simulink model "quadcopter_model_c_NewtonEuler"  (Simulink 10.1)
settings: Solver=ode3  StartTime=0.0  StopTime=100  FixedStep=inner_h  RelTol=1e-3  EnableMultiTasking=on
values from neighbouring files (symbols this model uses):
  A = [9.2e-07 9.1e-07 1.03e-06]    [dataset.mat]    (also in initiateVars.m = [0.92e-6; system_workspace.mat; system_workspace_ayk.mat)
  g = 9.81    [dataset.mat]    (also in initiateVars.m; system_workspace.mat; system_workspace_ayk.mat)
  I = eye(length(x_pred))    [MCKF.m]    (also in dataset.mat = [1.66e-05 1.66e-05 2.93e-05]; initiateVars.m = [1.66e-5; system_workspace.mat = [1.66e-05 1.66e-05 2.93e-05]; system_workspace_ayk.mat = [1.66e-05 1.66e-05 2.93e-05])
  m = 0.027    [dataset.mat]    (also in initiateVars.m; system_workspace.mat; system_workspace_ayk.mat)
libraries: sharedutil x1
settings Model: Creator=Daniel  LastModifiedBy=fethi
settings DataIOCC: LimitDataPoints=on  SaveFormat=Dataset
settings DebuggingCC: UnderspecifiedInitializationDetection=Simplified  MergeDetectMultiDrivingBlocksExec=error  AllowSymbolicDim=off  SFExecutionAtInitializationDiag=warning
settings HardwareCC: ProdBitPerPointer=64  ProdBitPerSizeT=64  ProdBitPerPtrDiffT=64  ProdLargestAtomicFloat=Float  ProdIntDivRoundTo=Zero  ProdEndianess=LittleEndian  ProdWordSize=64  ProdHWDeviceType=Intel->x86-64 (Windows64)
settings GRTTargetCC: CombineOutputUpdateFcns=on  GRTInterface=off

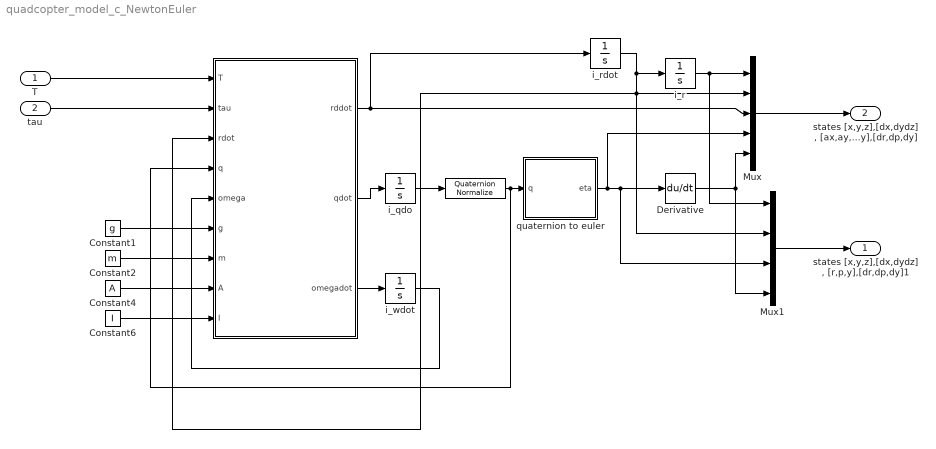
== system quadcopter_model_c_NewtonEuler ==
  T : Inport  PortDimensions=1
  tau : Inport  Port=2  PortDimensions=3
  " " : MATLAB Function  TreatAsAtomicUnit=on
  "  " : sharedutil/Quaternion Normalize  aMode=aMode
      settings: SourceProductBaseCode=AE,PW,MT,VE,VP
  Constant1 : Constant  Value=g
  Constant2 : Constant  Value=m
  Constant4 : Constant  Value=A
  Constant6 : Constant  Value=I
  Derivative : Derivative
  Mux : Mux  Inputs=5
  Mux1 : Mux
  i_qdo : Integrator  InitialCondition=[1; 0; 0; 0]
  i_r : Integrator  InitialCondition=[0.2 0.2 0]'
  i_rdot : Integrator  InitialCondition=[0; 0; 0]
  i_wdot : Integrator  InitialCondition=[0; 0; 0]
  quaternion to euler : MATLAB Function  TreatAsAtomicUnit=on
  "states [x,y,z],[dx,dydz], [r,p,y],[dr,dp,dy]1" : Outport  PortDimensions=12  VectorParamsAs1DForOutWhenUnconnected=off
  "states [x,y,z],[dx,dydz], [ax,ay,az],[r,p,y],[dr,dp,dy]" : Outport  Port=2  PortDimensions=15  VectorParamsAs1DForOutWhenUnconnected=off
  wires:
  " "/2(qdot) -> i_qdo/1
  " "/1(rddot) -> i_rdot/1, Mux/3
  i_r/1 -> Mux/1, Mux1/1
  T/1 -> " "/1(T)
  i_rdot/1 -> " "/3(rdot), Mux1/2, Mux/2, i_r/1
  tau/1 -> " "/2(tau)
  " "/3(omegadot) -> i_wdot/1
  Constant1/1 -> " "/6(g)
  Constant2/1 -> " "/7(m)
  Constant4/1 -> " "/8(A)
  Constant6/1 -> " "/9(I)
  i_wdot/1 -> " "/5(omega)
  i_qdo/1 -> "  "/1
  "  "/1 -> " "/4(q), quaternion to euler/1(q)
  quaternion to euler/1(eta) -> Mux/4, Mux1/3, Derivative/1
  Derivative/1 -> Mux/5, Mux1/4
  Mux/1 -> "states [x,y,z],[dx,dydz], [ax,ay,az],[r,p,y],[dr,dp,dy]"/1
  Mux1/1 -> "states [x,y,z],[dx,dydz], [r,p,y],[dr,dp,dy]1"/1

== matlab function   ==
  data: T input double; tau input double; rddot output double; rdot input double; q input double; omega input double; qdot output double; g input double; m input double; A input double; I input double; omegadot output double
function [ rddot,qdot,omegadot] = quad_acceleration(T, tau, rdot, q, omega, g, m, A, I)

    qw = q(1); qx = q(2); qy = q(3); qz = q(4); qv = q(2:4);
    omegaw = 0; omegav = omega;
    
    % Gravity acceleration
    Ga = -g * [0; 0; 1];

    % TODO write rotation
    angM = [2*(qx*qz + qw*qy);
            2*(qy*qz - qw*qx);
            qw.^2 - qx.^2 - qy.^2 + qz.^2];

    Ta = (T/m) .* angM;

    % Drag
    Aa = -1/m * diag(A) * rdot;
    rddot = Ga + Ta + Aa;
    
    % Define the C-matrix as (19)
    J = diag(I);
    qcross = [0, -qz, qy; qz, 0, -qx; -qy, qx, 0];
    qdot = 0.5.*(eye(4)*qw  + [0, -qv';qv, qcross])*[0; omegav];
    omegadot = J\(tau - cross(omegav, J*omegav));
    
%     R = [qw^2+qx^2+qy^2+qz^2, 2*(qx*qy-qw*qz)    , 2*(qx*qz+qw*qy);
%          2*(qx*qy+qw*qz)    , qw^2-qx^2+qy^2-qz^2, 2*(qy*qz-qw*qx);
%          2*(qx*qz-qw*qy)    , 2*(qy*qz+qw*qx)    , qw^2-qx^2-qy^2+qz^2];

end

== matlab function quaternion to euler ==
  data: q input double; eta output double
function eta = fcn(q)
%#codegen
phi = atan2(2*(q(1)*q(2) + q(3)*q(4)), q(1)^2 - q(2)^2 - q(3)^2 + q(4)^2);
theta = asin(2*(q(1)*q(3) - q(4)*q(2)));
psi = atan2(2*(q(1)*q(4) + q(2)*q(3)), q(1)^2 + q(2)^2 - q(3)^2 - q(4)^2);
eta = [phi;theta;psi];
